simulink model "lab4_sim3"  (R2022b)
settings: Solver=VariableStepAuto  StartTime=0.0  StopTime=time  RelTol=1e-3
values from neighbouring files (symbols this model uses):
  B = 0.165    [script.m]
  goal_x = x_finish(i)    [script.m]
  goal_y = y_finish(i)    [script.m]
  J = 0.0023766912    [script.m]
  k_e = 0.5447005537429133    (= 0.544700553743)    [script.m]
  k_m = 0.5447005537429133    (= 0.544700553743)    [script.m]
  K_r = 35    [script.m]
  K_s = 20    [script.m]
  L = 0.0047    [script.m]
  r = 0.021    [script.m]
  R = 12.263574138575136    (= 12.2635741386)    [script.m]
  th0 = sim_data.th0.Data(end)    [script.m]
  x0 = sim_data.x.Data(end)    [script.m]
  y0 = sim_data.y.Data(end)    [script.m]
settings Model: Creator=LaKeR  LastModifiedBy=LaKeR

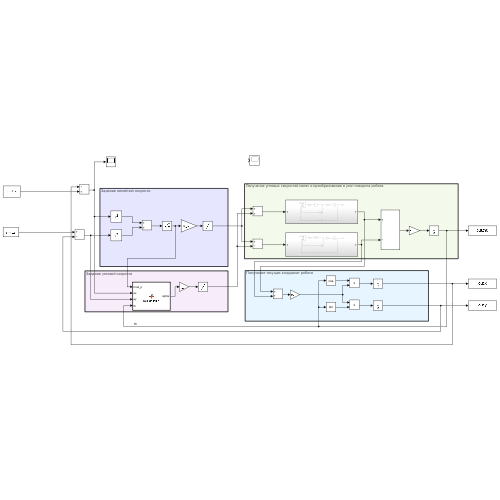
[thumbnail: Simulink's stored preview of the top-level diagram]
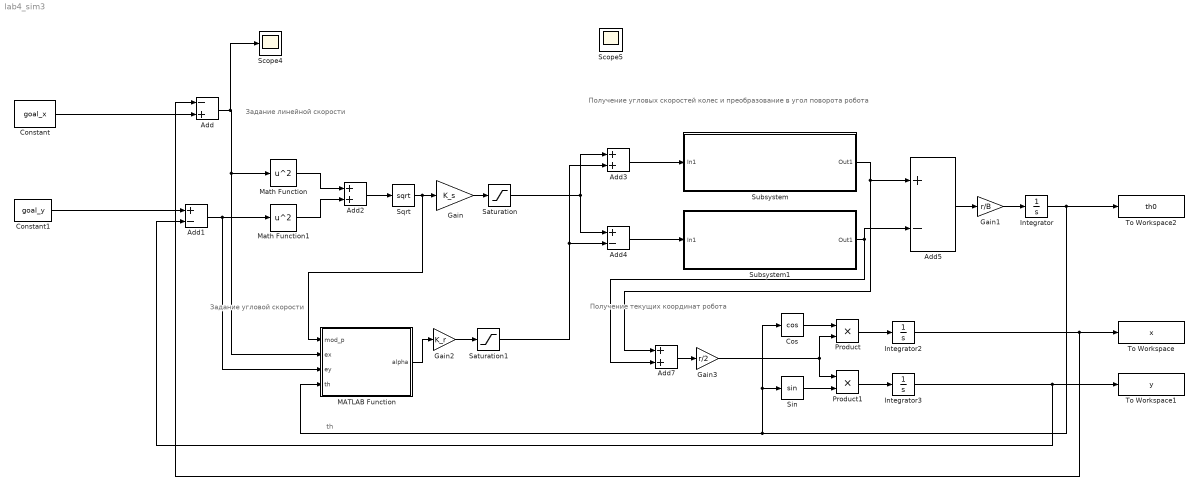
== system lab4_sim3 ==
  note: th
  note: Получение текущих координат робота
  note: Задание угловой скорости
  note: Получение угловых скоростей колес и преобразование в угол поворота робота
  note: Задание линейной скорости
  Add : Sum  Inputs=-+
  Add1 : Sum  Inputs=+-
  Add2 : Sum
  Add3 : Sum
  Add4 : Sum  Inputs=+-
  Add5 : Sum  Inputs=+-
  Add7 : Sum
  Constant : Constant  Value=goal_x
  Constant1 : Constant  Value=goal_y
  Cos : Trigonometry  Operator=cos
  Gain : Gain  Gain=K_s
  Gain1 : Gain  Gain=r/B
  Gain2 : Gain  Gain=K_r
  Gain3 : Gain  Gain=r/2
  Integrator : Integrator  InitialCondition=th0
  Integrator2 : Integrator  InitialCondition=x0
  Integrator3 : Integrator  InitialCondition=y0
  MATLAB Function : MATLAB Function  TreatAsAtomicUnit=on
  Math Function : Math  Operator=square
  Math Function1 : Math  Operator=square
  Product : Product
  Product1 : Product
  Saturation : Saturate
  Saturation1 : Saturate
  Scope4 : Scope
  Scope5 : Scope
  Sin : Trigonometry
  Sqrt : Sqrt
  Subsystem : Subsystem
  Subsystem1 : Subsystem
  To Workspace : ToWorkspace  VariableName=x  SaveFormat=Timeseries  SampleTime=-1
  To Workspace1 : ToWorkspace  VariableName=y  SaveFormat=Timeseries  SampleTime=-1
  To Workspace2 : ToWorkspace  VariableName=th0  SaveFormat=Timeseries  SampleTime=-1
  wires:
  Subsystem1/1(Out1) -> Add5/2, Add7/2
  Cos/1 -> Product/1
  Gain1/1 -> Integrator/1
  MATLAB Function/1(alpha) -> Gain2/1
  Product/1 -> Integrator2/1
  Integrator3/1 -> Add1/2, To Workspace1/1
  Integrator2/1 -> Add/1, To Workspace/1
  Product1/1 -> Integrator3/1
  Gain/1 -> Saturation/1
  Add7/1 -> Gain3/1
  Gain3/1 -> Product/2, Product1/1
  Sqrt/1 -> MATLAB Function/1(mod_p), Gain/1
  Subsystem/1(Out1) -> Add5/1, Add7/1
  Add3/1 -> Subsystem/1(In1)
  Add4/1 -> Subsystem1/1(In1)
  Gain2/1 -> Saturation1/1
  Add1/1 -> MATLAB Function/3(ey), Math Function1/1
  Saturation1/1 -> Add3/2, Add4/2
  Add2/1 -> Sqrt/1
  Sin/1 -> Product1/2
  Add/1 -> Scope4/1, MATLAB Function/2(ex), Math Function/1
  Math Function1/1 -> Add2/2
  Saturation/1 -> Add4/1, Add3/1
  Math Function/1 -> Add2/1
  Add5/1 -> Gain1/1
  Constant1/1 -> Add1/1
  Constant/1 -> Add/2
  Integrator/1 -> To Workspace2/1, MATLAB Function/4(th), Cos/1, Sin/1

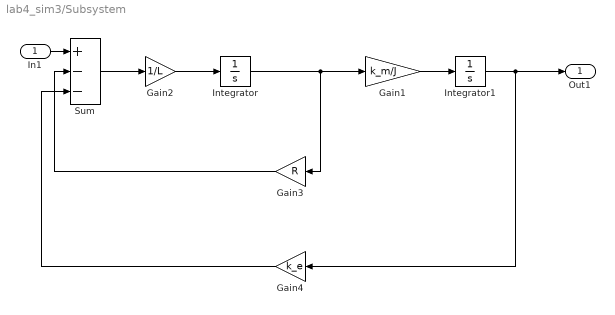
== system lab4_sim3/Subsystem ==
  In1 : Inport
  Gain1 : Gain  Gain=k_m/J
  Gain2 : Gain  Gain=1/L
  Gain3 : Gain  Gain=R
  Gain4 : Gain  Gain=k_e
  Integrator : Integrator
  Integrator1 : Integrator
  Sum : Sum  Inputs=+--
  Out1 : Outport
  wires:
  Gain1/1 -> Integrator1/1
  Integrator/1 -> Gain3/1, Gain1/1
  Gain4/1 -> Sum/3
  Integrator1/1 -> Gain4/1, Out1/1
  In1/1 -> Sum/1
  Sum/1 -> Gain2/1
  Gain2/1 -> Integrator/1
  Gain3/1 -> Sum/2

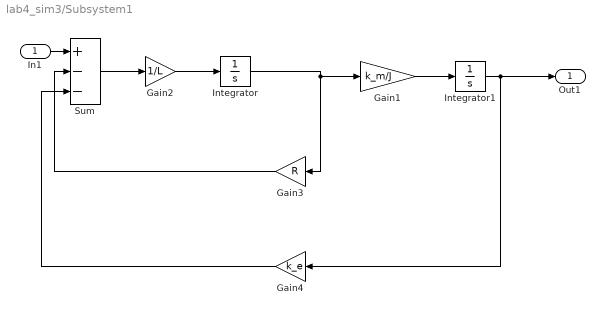
== system lab4_sim3/Subsystem1 ==
  In1 : Inport
  Gain1 : Gain  Gain=k_m/J
  Gain2 : Gain  Gain=1/L
  Gain3 : Gain  Gain=R
  Gain4 : Gain  Gain=k_e
  Integrator : Integrator
  Integrator1 : Integrator
  Sum : Sum  Inputs=+--
  Out1 : Outport
  wires:
  Gain1/1 -> Integrator1/1
  Integrator/1 -> Gain3/1, Gain1/1
  Gain4/1 -> Sum/3
  Integrator1/1 -> Out1/1, Gain4/1
  In1/1 -> Sum/1
  Sum/1 -> Gain2/1
  Gain2/1 -> Integrator/1
  Gain3/1 -> Sum/2

== matlab function lab4_sim3/MATLAB Function ==
  data: mod_p input; ex input; ey input; th input; alpha output
function alpha = myFunction(mod_p, ex, ey,  th)

A_1 = (cos(th) * ey - sin(th) * ex) / mod_p;
CS = (cos(th) * ex + sin(th) * ey) / mod_p;

if CS < 0
    A_1 = 1;
end

alpha = A_1;

end
